simulink model "Zone_1_Zone_2_Thyristor_240Hz_R2022b"  (R2022b)
settings: Solver=FixedStepDiscrete  StartTime=0.0  StopTime=5  FixedStep=Ts  RelTol=1e-3  EnableMultiTasking=on
undefined symbols (not defined in the file or in its folder): DiscIntNeverNeededParam, GABDA, GABDB, GBBDA, GBBDB, GPPMA, GPPMB, GPPMC, SADA, SADB, SADC, SADD, SBDA, SBDB, SBDC, SCDA, SCDB, SCDC, SCDD, SDDA, SDDB, SDDC, SDDD, SDDE, TsELEC
libraries: nesl_utility x70, fl_lib x60, ee_lib x44, eeThyristorSixPulseGenerator x2, spsPowerLib x2, eeSinusoidalMeasurement x2
(part 3 of 3)

== system Zone_1_Zone_2_Thyristor_240Hz_R2022b/Subsystem16 ==
  Inductor1 : fl_lib/Electrical/Electrical Elements/Inductor  l=5.32e-6/2 H  r=0.32e-3/2 Ohm  g=0 1/Ohm  i_specify=off  i_priority=None  i=0 A  i_nominal_specify=off  i_nominal_unit=A  i_nominal_value=1  v_specify=off  v_priority=None  v=0 V  v_nominal_specify=off  v_nominal_unit=V  v_nominal_value=1  i_L_specify=off  i_L_priority=High  i_L=0 A  i_L_nominal_specify=off  i_L_nominal_unit=A  i_L_nominal_value=1
  Inductor2 : fl_lib/Electrical/Electrical Elements/Inductor  l=5.32e-6/2 H  r=0.32e-3/2 Ohm  g=0 1/Ohm  i_specify=off  i_priority=None  i=0 A  i_nominal_specify=off  i_nominal_unit=A  i_nominal_value=1  v_specify=off  v_priority=None  v=0 V  v_nominal_specify=off  v_nominal_unit=V  v_nominal_value=1  i_L_specify=off  i_L_priority=High  i_L=0 A  i_L_nominal_specify=off  i_L_nominal_unit=A  i_L_nominal_value=1
  "+ " : PMIOPort  Side=Left
  + : PMIOPort  Port=2  Side=Right
  - : PMIOPort  Port=3  Side=Left
  "- " : PMIOPort  Port=4  Side=Right
  connections:
  Inductor1/RConn1 -- "- "/RConn1
  Inductor2/RConn1 -- +/RConn1
  Inductor2/LConn1 -- "+ "/RConn1
  Inductor1/LConn1 -- -/RConn1

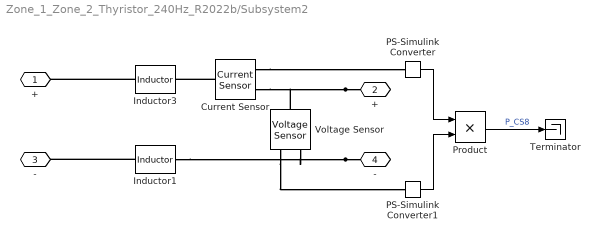
== system Zone_1_Zone_2_Thyristor_240Hz_R2022b/Subsystem2 ==
  Current Sensor : fl_lib/Electrical/Electrical Sensors/Current Sensor
  Inductor1 : fl_lib/Electrical/Electrical Elements/Inductor  l=5e-6/2 H  r=0.2e-3/2 Ohm  g=0 1/Ohm  i_specify=off  i_priority=None  i=0 A  i_nominal_specify=off  i_nominal_unit=A  i_nominal_value=1  v_specify=off  v_priority=None  v=0 V  v_nominal_specify=off  v_nominal_unit=V  v_nominal_value=1  i_L_specify=off  i_L_priority=High  i_L=0 A  i_L_nominal_specify=off  i_L_nominal_unit=A  i_L_nominal_value=1
  Inductor3 : fl_lib/Electrical/Electrical Elements/Inductor  l=5e-6/2 H  r=0.2e-3/2 Ohm  g=0 1/Ohm  i_specify=off  i_priority=None  i=0 A  i_nominal_specify=off  i_nominal_unit=A  i_nominal_value=1  v_specify=off  v_priority=None  v=0 V  v_nominal_specify=off  v_nominal_unit=V  v_nominal_value=1  i_L_specify=off  i_L_priority=High  i_L=0 A  i_L_nominal_specify=off  i_L_nominal_unit=A  i_L_nominal_value=1
  PS-Simulink Converter : nesl_utility/PS-Simulink Converter  PhysicalDomain=network_engine_domain  SubClassName=ps_output  LeftPortType=input  RightPortType=output  PseudoPeriodic=off  Frequencies=[]  VectorFormat=1-D array  Unit=inherit  AffineConversion=off
  PS-Simulink Converter1 : nesl_utility/PS-Simulink Converter  PhysicalDomain=network_engine_domain  SubClassName=ps_output  LeftPortType=input  RightPortType=output  PseudoPeriodic=off  Frequencies=[]  VectorFormat=1-D array  Unit=inherit  AffineConversion=off
  Product : Product
  Terminator : Terminator
  Voltage Sensor : fl_lib/Electrical/Electrical Sensors/Voltage Sensor
  "+ " : PMIOPort  Side=Left
  + : PMIOPort  Port=2  Side=Right
  - : PMIOPort  Port=3  Side=Left
  "- " : PMIOPort  Port=4  Side=Right
  wires:
  PS-Simulink Converter1/1 -> Product/2
  PS-Simulink Converter/1 -> Product/1
  Product/1 -> Terminator/1  "P_CS8"
  connections:
  Current Sensor/RConn1 -- PS-Simulink Converter/LConn1
  Voltage Sensor/RConn1 -- PS-Simulink Converter1/LConn1
  "- "/RConn1 -- Voltage Sensor/RConn2 -- Inductor1/RConn1
  +/RConn1 -- Voltage Sensor/LConn1 -- Current Sensor/RConn2
  Current Sensor/LConn1 -- Inductor3/RConn1
  Inductor3/LConn1 -- "+ "/RConn1
  Inductor1/LConn1 -- -/RConn1

== system Zone_1_Zone_2_Thyristor_240Hz_R2022b/Subsystem3 ==
  Inductor1 : fl_lib/Electrical/Electrical Elements/Inductor  l=2.63e-6/2 H  r=0.16e-3/2 Ohm  g=0 1/Ohm  i_specify=off  i_priority=None  i=0 A  i_nominal_specify=off  i_nominal_unit=A  i_nominal_value=1  v_specify=off  v_priority=None  v=0 V  v_nominal_specify=off  v_nominal_unit=V  v_nominal_value=1  i_L_specify=off  i_L_priority=High  i_L=0 A  i_L_nominal_specify=off  i_L_nominal_unit=A  i_L_nominal_value=1
  Inductor3 : fl_lib/Electrical/Electrical Elements/Inductor  l=2.63e-6/2 H  r=0.16e-3/2 Ohm  g=0 1/Ohm  i_specify=off  i_priority=None  i=0 A  i_nominal_specify=off  i_nominal_unit=A  i_nominal_value=1  v_specify=off  v_priority=None  v=0 V  v_nominal_specify=off  v_nominal_unit=V  v_nominal_value=1  i_L_specify=off  i_L_priority=High  i_L=0 A  i_L_nominal_specify=off  i_L_nominal_unit=A  i_L_nominal_value=1
  "+ " : PMIOPort  Side=Left
  + : PMIOPort  Port=2  Side=Right
  - : PMIOPort  Port=3  Side=Left
  "- " : PMIOPort  Port=4  Side=Right
  connections:
  Inductor1/RConn1 -- "- "/RConn1
  Inductor3/RConn1 -- +/RConn1
  Inductor3/LConn1 -- "+ "/RConn1
  Inductor1/LConn1 -- -/RConn1

== system Zone_1_Zone_2_Thyristor_240Hz_R2022b/Subsystem4 ==
  In1 : Inport
  Demux1 : Demux  Outputs=[9 1 1]
  Terminator : Terminator
  breaker status : Subsystem
  tag scope: Z1_Efd=global
  wires:
  Demux1/1 -> breaker status/1(In1)  "breakers"
  Demux1/3 -> Terminator/1
  Demux1/2 -> [Z1_Efd]  "Efd"
  In1/1 -> Demux1/1

== system Zone_1_Zone_2_Thyristor_240Hz_R2022b/Subsystem5 ==
  Inductor1 : fl_lib/Electrical/Electrical Elements/Inductor  l=5.32e-6/2 H  r=0.32e-3/2 Ohm  g=0 1/Ohm  i_specify=off  i_priority=None  i=0 A  i_nominal_specify=off  i_nominal_unit=A  i_nominal_value=1  v_specify=off  v_priority=None  v=0 V  v_nominal_specify=off  v_nominal_unit=V  v_nominal_value=1  i_L_specify=off  i_L_priority=High  i_L=0 A  i_L_nominal_specify=off  i_L_nominal_unit=A  i_L_nominal_value=1
  Inductor2 : fl_lib/Electrical/Electrical Elements/Inductor  l=5.32e-6/2 H  r=0.32e-3/2 Ohm  g=0 1/Ohm  i_specify=off  i_priority=None  i=0 A  i_nominal_specify=off  i_nominal_unit=A  i_nominal_value=1  v_specify=off  v_priority=None  v=0 V  v_nominal_specify=off  v_nominal_unit=V  v_nominal_value=1  i_L_specify=off  i_L_priority=High  i_L=0 A  i_L_nominal_specify=off  i_L_nominal_unit=A  i_L_nominal_value=1
  "+ " : PMIOPort  Side=Left
  + : PMIOPort  Port=2  Side=Right
  - : PMIOPort  Port=3  Side=Left
  "- " : PMIOPort  Port=4  Side=Right
  connections:
  Inductor1/LConn1 -- -/RConn1
  Inductor2/LConn1 -- "+ "/RConn1
  Inductor2/RConn1 -- +/RConn1
  Inductor1/RConn1 -- "- "/RConn1

== system Zone_1_Zone_2_Thyristor_240Hz_R2022b/Subsystem6 ==
  In1 : Inport
  Demux2 : Demux  Outputs=[14 1 1 1]
  Terminator1 : Terminator
  breaker status1 : Subsystem
  tag scope: PMM=global, Z2_Efd=global
  wires:
  Demux2/1 -> breaker status1/1(In1)  "breakers"
  Demux2/3 -> Terminator1/1
  Demux2/4 -> [PMM]
  Demux2/2 -> [Z2_Efd]  "Efd"
  In1/1 -> Demux2/1

== system Zone_1_Zone_2_Thyristor_240Hz_R2022b/Subsystem7 ==
  Simulink-PS Converter : nesl_utility/Simulink-PS Converter  PhysicalDomain=network_engine_domain  SubClassName=ps_input  LeftPortType=input  RightPortType=output  PseudoPeriodic=off  Frequencies=[]  NoiseDistribution=none  NoiseParameters=[]  Unit=1  AffineConversion=off  FilteringAndDerivatives=provide  SimscapeFilterOrder=1  InputFilterTimeConstant=0.001  UdotUserProvided=0
  Variable Resistor : fl_lib/Electrical/Electrical Elements/Variable Resistor  Rmin=0 Ohm  i_specify=off  i_priority=None  i=0 A  i_nominal_specify=off  i_nominal_unit=A  i_nominal_value=1  v_specify=off  v_priority=None  v=0 V  v_nominal_specify=off  v_nominal_unit=V  v_nominal_value=1
  + : PMIOPort  Side=Left
  - : PMIOPort  Port=2  Side=Left
  wires:
  [PMM] -> Simulink-PS Converter/1
  connections:
  Simulink-PS Converter/RConn1 -- Variable Resistor/LConn1
  Variable Resistor/LConn2 -- +/RConn1
  Variable Resistor/RConn1 -- -/RConn1

== system Zone_1_Zone_2_Thyristor_240Hz_R2022b/Subsystem8 ==
  Inductor1 : fl_lib/Electrical/Electrical Elements/Inductor  l=2.63e-6/2 H  r=0.16e-3/2 Ohm  g=0 1/Ohm  i_specify=off  i_priority=None  i=0 A  i_nominal_specify=off  i_nominal_unit=A  i_nominal_value=1  v_specify=off  v_priority=None  v=0 V  v_nominal_specify=off  v_nominal_unit=V  v_nominal_value=1  i_L_specify=off  i_L_priority=High  i_L=0 A  i_L_nominal_specify=off  i_L_nominal_unit=A  i_L_nominal_value=1
  Inductor3 : fl_lib/Electrical/Electrical Elements/Inductor  l=2.63e-6/2 H  r=0.16e-3/2 Ohm  g=0 1/Ohm  i_specify=off  i_priority=None  i=0 A  i_nominal_specify=off  i_nominal_unit=A  i_nominal_value=1  v_specify=off  v_priority=None  v=0 V  v_nominal_specify=off  v_nominal_unit=V  v_nominal_value=1  i_L_specify=off  i_L_priority=High  i_L=0 A  i_L_nominal_specify=off  i_L_nominal_unit=A  i_L_nominal_value=1
  "+ " : PMIOPort  Side=Left
  + : PMIOPort  Port=2  Side=Right
  - : PMIOPort  Port=3  Side=Left
  "- " : PMIOPort  Port=4  Side=Right
  connections:
  Inductor1/LConn1 -- -/RConn1
  Inductor3/LConn1 -- "+ "/RConn1
  Inductor3/RConn1 -- +/RConn1
  Inductor1/RConn1 -- "- "/RConn1

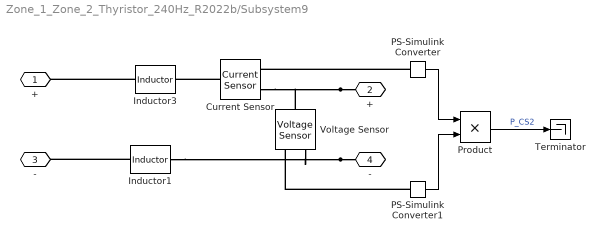
== system Zone_1_Zone_2_Thyristor_240Hz_R2022b/Subsystem9 ==
  Current Sensor : fl_lib/Electrical/Electrical Sensors/Current Sensor
  Inductor1 : fl_lib/Electrical/Electrical Elements/Inductor  l=3.47e-6/2 H  r=0.21e-3/2 Ohm  g=0 1/Ohm  i_specify=off  i_priority=None  i=0 A  i_nominal_specify=off  i_nominal_unit=A  i_nominal_value=1  v_specify=off  v_priority=None  v=0 V  v_nominal_specify=off  v_nominal_unit=V  v_nominal_value=1  i_L_specify=off  i_L_priority=High  i_L=0 A  i_L_nominal_specify=off  i_L_nominal_unit=A  i_L_nominal_value=1
  Inductor3 : fl_lib/Electrical/Electrical Elements/Inductor  l=3.47e-6/2 H  r=0.21e-3/2 Ohm  g=0 1/Ohm  i_specify=off  i_priority=None  i=0 A  i_nominal_specify=off  i_nominal_unit=A  i_nominal_value=1  v_specify=off  v_priority=None  v=0 V  v_nominal_specify=off  v_nominal_unit=V  v_nominal_value=1  i_L_specify=off  i_L_priority=High  i_L=0 A  i_L_nominal_specify=off  i_L_nominal_unit=A  i_L_nominal_value=1
  PS-Simulink Converter : nesl_utility/PS-Simulink Converter  PhysicalDomain=network_engine_domain  SubClassName=ps_output  LeftPortType=input  RightPortType=output  PseudoPeriodic=off  Frequencies=[]  VectorFormat=1-D array  Unit=inherit  AffineConversion=off
  PS-Simulink Converter1 : nesl_utility/PS-Simulink Converter  PhysicalDomain=network_engine_domain  SubClassName=ps_output  LeftPortType=input  RightPortType=output  PseudoPeriodic=off  Frequencies=[]  VectorFormat=1-D array  Unit=inherit  AffineConversion=off
  Product : Product
  Terminator : Terminator
  Voltage Sensor : fl_lib/Electrical/Electrical Sensors/Voltage Sensor
  "+ " : PMIOPort  Side=Left
  + : PMIOPort  Port=2  Side=Right
  - : PMIOPort  Port=3  Side=Left
  "- " : PMIOPort  Port=4  Side=Right
  wires:
  Product/1 -> Terminator/1  "P_CS2"
  PS-Simulink Converter1/1 -> Product/2
  PS-Simulink Converter/1 -> Product/1
  connections:
  PS-Simulink Converter1/LConn1 -- Voltage Sensor/RConn1
  PS-Simulink Converter/LConn1 -- Current Sensor/RConn1
  +/RConn1 -- Voltage Sensor/LConn1 -- Current Sensor/RConn2
  Current Sensor/LConn1 -- Inductor3/RConn1
  "- "/RConn1 -- Voltage Sensor/RConn2 -- Inductor1/RConn1
  Inductor1/LConn1 -- -/RConn1
  Inductor3/LConn1 -- "+ "/RConn1

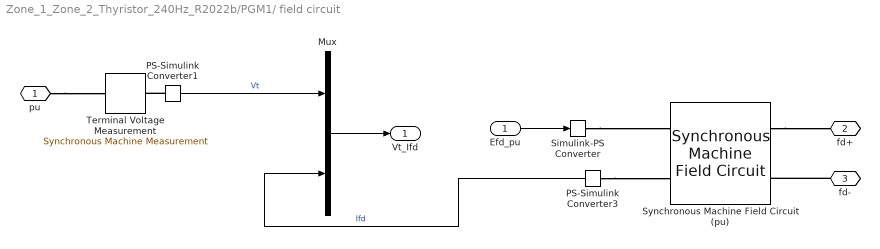
== system Zone_1_Zone_2_Thyristor_240Hz_R2022b/PGM1/ field circuit ==
  Efd_pu : Inport
  Mux : Mux  Inputs=2
  PS-Simulink Converter1 : nesl_utility/PS-Simulink Converter  PhysicalDomain=network_engine_domain  SubClassName=ps_output  LeftPortType=input  RightPortType=output  PseudoPeriodic=off  Frequencies=[]  VectorFormat=1-D array  Unit=inherit  AffineConversion=off
  PS-Simulink Converter3 : nesl_utility/PS-Simulink Converter  PhysicalDomain=network_engine_domain  SubClassName=ps_output  LeftPortType=input  RightPortType=output  PseudoPeriodic=off  Frequencies=[]  VectorFormat=1-D array  Unit=inherit  AffineConversion=off
  Simulink-PS Converter : nesl_utility/Simulink-PS Converter  PhysicalDomain=network_engine_domain  SubClassName=ps_input  LeftPortType=input  RightPortType=output  PseudoPeriodic=off  Frequencies=[]  NoiseDistribution=none  NoiseParameters=[]  Unit=1  AffineConversion=off  FilteringAndDerivatives=zero  SimscapeFilterOrder=1  InputFilterTimeConstant=0.001  UdotUserProvided=0
  Synchronous Machine Field Circuit (pu) : ee_lib/Electromechanical/Synchronous/Synchronous Machine Field Circuit  unit_option=ee.enum.unit.pu  SRated=45e6 V*A  FRated=240 Hz  fieldCircuitParameterization_option=ee.enum.sm.fieldparameterization.current  baseEfd=92.95 V  baseIfd=200 A  parameterization_option=ee.enum.sm.parameterization.standard  Ladu=1.66  Rfd=0.0006  Xl=0.08  Xd=1.352  Xdd=0.296  Xddd=0.148  d_option=ee.enum.circuit.open  Td0d=4.141 s  Tdd=1.3260 s  Td0dd=0.027 s  Tddd=0.0230 s
      settings: LogSimulationData=on  InternalSimscapePortConfiguration="{\"Bottom\":[],\"Left\":[{\"id\":\"Efd_pu\",\"label\":\"Efd_pu\",\"type\":\"input\"},{\"id\":\"Ifd_pu\",\"label\":\"Ifd_pu\",\"type\":\"output\"}],\"Right\":[{\"id\":\"fd_p\",\"label\":\"fd+\",\"type\":\"foundation.electrical.electrical\"},{\"id\":\"fd_n\",\"label\":\"fd-\",\"type\":\"foundation.electrical.electrical\"}],\"Top\":[]}"
  Terminal Voltage Measurement : ee_lib/Electromechanical/Synchronous/Synchronous Machine Measurement  output_idx=14
      settings: LogSimulationData=on  InternalSimscapePortConfiguration="{\"Bottom\":[],\"Left\":[{\"id\":\"pu_input\",\"label\":\"pu\",\"type\":\"input\"}],\"Right\":[{\"id\":\"pu_output\",\"label\":\"o\",\"type\":\"output\"}],\"Top\":[]}"
  pu : PMIOPort  Side=Left
  fd+ : PMIOPort  Port=2  Side=Right
  fd- : PMIOPort  Port=3  Side=Right
  Vt_Ifd : Outport
  wires:
  Mux/1 -> Vt_Ifd/1
  PS-Simulink Converter3/1 -> Mux/2  "Ifd"
  PS-Simulink Converter1/1 -> Mux/1  "Vt"
  Efd_pu/1 -> Simulink-PS Converter/1
  connections:
  PS-Simulink Converter1/LConn1 -- Terminal Voltage Measurement/RConn1
  pu/RConn1 -- Terminal Voltage Measurement/LConn1
  Simulink-PS Converter/RConn1 -- Synchronous Machine Field Circuit (pu)/LConn1
  PS-Simulink Converter3/LConn1 -- Synchronous Machine Field Circuit (pu)/LConn2
  Synchronous Machine Field Circuit (pu)/RConn1 -- fd+/RConn1
  fd-/RConn1 -- Synchronous Machine Field Circuit (pu)/RConn2

== system Zone_1_Zone_2_Thyristor_240Hz_R2022b/PGM1/Gate driver ==
  S : Inport
  Demux : Demux  Outputs=6
  Simulink-PS Converter{,1..5} (6 alike) : nesl_utility/Simulink-PS Converter  PhysicalDomain=network_engine_domain  SubClassName=ps_input  LeftPortType=input  RightPortType=output  PseudoPeriodic=off  Frequencies=[]  NoiseDistribution=none  NoiseParameters=[]  Unit=1  AffineConversion=off  FilteringAndDerivatives=zero  SimscapeFilterOrder=1  InputFilterTimeConstant=0.001  UdotUserProvided=0
  Six-Pulse Gate Multiplexer : ee_lib/Semiconductors & Converters/Converters/Six-Pulse Gate Multiplexer  port_option=ee.enum.controlport.ps
  G : PMIOPort  Side=Right
  wires:
  Demux/1 -> Simulink-PS Converter/1
  Demux/5 -> Simulink-PS Converter4/1
  Demux/2 -> Simulink-PS Converter1/1
  Demux/4 -> Simulink-PS Converter3/1
  S/1 -> Demux/1
  Demux/3 -> Simulink-PS Converter2/1
  Demux/6 -> Simulink-PS Converter5/1
  connections:
  Six-Pulse Gate Multiplexer/RConn1 -- G/RConn1
  Simulink-PS Converter4/RConn1 -- Six-Pulse Gate Multiplexer/LConn5
  Simulink-PS Converter/RConn1 -- Six-Pulse Gate Multiplexer/LConn1
  Simulink-PS Converter3/RConn1 -- Six-Pulse Gate Multiplexer/LConn4
  Simulink-PS Converter2/RConn1 -- Six-Pulse Gate Multiplexer/LConn3
  Simulink-PS Converter1/RConn1 -- Six-Pulse Gate Multiplexer/LConn2
  Simulink-PS Converter5/RConn1 -- Six-Pulse Gate Multiplexer/LConn6

== system Zone_1_Zone_2_Thyristor_240Hz_R2022b/PGM1/Sensing current ==
  Current Sensor : ee_lib/Sensors & Transducers/Current Sensor (Three-Phase)
  PS-Simulink Converter : nesl_utility/PS-Simulink Converter  PhysicalDomain=network_engine_domain  SubClassName=ps_output  LeftPortType=input  RightPortType=output  PseudoPeriodic=off  Frequencies=[]  VectorFormat=1-D array  Unit=A  AffineConversion=off
  1~ : PMIOPort  Side=Left
  2~ : PMIOPort  Port=2  Side=Right
  tag scope: Iabc1=global
  wires:
  PS-Simulink Converter/1 -> [Iabc1]
  connections:
  2~/RConn1 -- Current Sensor/RConn2
  PS-Simulink Converter/LConn1 -- Current Sensor/RConn1
  Current Sensor/LConn1 -- 1~/RConn1

== system Zone_1_Zone_2_Thyristor_240Hz_R2022b/PGM1/Sensing voltage ==
  PS-Simulink Converter : nesl_utility/PS-Simulink Converter  PhysicalDomain=network_engine_domain  SubClassName=ps_output  LeftPortType=input  RightPortType=output  PseudoPeriodic=off  Frequencies=[]  VectorFormat=1-D array  Unit=V  AffineConversion=off
  Phase Voltage Sensor : ee_lib/Sensors & Transducers/Phase Voltage Sensor (Three-Phase)
  ~2 : PMIOPort  Side=Right
  ~1 : PMIOPort  Port=2  Side=Left
  tag scope: Vabc1=global
  wires:
  PS-Simulink Converter/1 -> [Vabc1]
  connections:
  Phase Voltage Sensor/LConn1 -- ~1/RConn1
  Phase Voltage Sensor/RConn2 -- ~2/RConn1
  PS-Simulink Converter/LConn1 -- Phase Voltage Sensor/RConn1

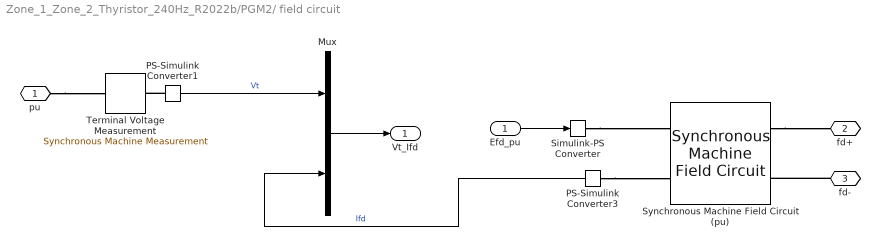
== system Zone_1_Zone_2_Thyristor_240Hz_R2022b/PGM2/ field circuit ==
  Efd_pu : Inport
  Mux : Mux  Inputs=2
  PS-Simulink Converter1 : nesl_utility/PS-Simulink Converter  PhysicalDomain=network_engine_domain  SubClassName=ps_output  LeftPortType=input  RightPortType=output  PseudoPeriodic=off  Frequencies=[]  VectorFormat=1-D array  Unit=inherit  AffineConversion=off
  PS-Simulink Converter3 : nesl_utility/PS-Simulink Converter  PhysicalDomain=network_engine_domain  SubClassName=ps_output  LeftPortType=input  RightPortType=output  PseudoPeriodic=off  Frequencies=[]  VectorFormat=1-D array  Unit=inherit  AffineConversion=off
  Simulink-PS Converter : nesl_utility/Simulink-PS Converter  PhysicalDomain=network_engine_domain  SubClassName=ps_input  LeftPortType=input  RightPortType=output  PseudoPeriodic=off  Frequencies=[]  NoiseDistribution=none  NoiseParameters=[]  Unit=1  AffineConversion=off  FilteringAndDerivatives=zero  SimscapeFilterOrder=1  InputFilterTimeConstant=0.001  UdotUserProvided=0
  Synchronous Machine Field Circuit (pu) : ee_lib/Electromechanical/Synchronous/Synchronous Machine Field Circuit  unit_option=ee.enum.unit.pu  SRated=45e6 V*A  FRated=240 Hz  fieldCircuitParameterization_option=ee.enum.sm.fieldparameterization.current  baseEfd=92.95 V  baseIfd=200 A  parameterization_option=ee.enum.sm.parameterization.standard  Ladu=1.66  Rfd=0.0006  Xl=0.08  Xd=1.352  Xdd=0.296  Xddd=0.148  d_option=ee.enum.circuit.open  Td0d=4.141 s  Tdd=1.3260 s  Td0dd=0.027 s  Tddd=0.0230 s
      settings: LogSimulationData=on  InternalSimscapePortConfiguration="{\"Bottom\":[],\"Left\":[{\"id\":\"Efd_pu\",\"label\":\"Efd_pu\",\"type\":\"input\"},{\"id\":\"Ifd_pu\",\"label\":\"Ifd_pu\",\"type\":\"output\"}],\"Right\":[{\"id\":\"fd_p\",\"label\":\"fd+\",\"type\":\"foundation.electrical.electrical\"},{\"id\":\"fd_n\",\"label\":\"fd-\",\"type\":\"foundation.electrical.electrical\"}],\"Top\":[]}"
  Terminal Voltage Measurement : ee_lib/Electromechanical/Synchronous/Synchronous Machine Measurement  output_idx=14
      settings: LogSimulationData=on  InternalSimscapePortConfiguration="{\"Bottom\":[],\"Left\":[{\"id\":\"pu_input\",\"label\":\"pu\",\"type\":\"input\"}],\"Right\":[{\"id\":\"pu_output\",\"label\":\"o\",\"type\":\"output\"}],\"Top\":[]}"
  pu : PMIOPort  Side=Left
  fd+ : PMIOPort  Port=2  Side=Right
  fd- : PMIOPort  Port=3  Side=Right
  Vt_Ifd : Outport
  wires:
  Efd_pu/1 -> Simulink-PS Converter/1
  PS-Simulink Converter1/1 -> Mux/1  "Vt"
  PS-Simulink Converter3/1 -> Mux/2  "Ifd"
  Mux/1 -> Vt_Ifd/1
  connections:
  fd-/RConn1 -- Synchronous Machine Field Circuit (pu)/RConn2
  Synchronous Machine Field Circuit (pu)/RConn1 -- fd+/RConn1
  PS-Simulink Converter3/LConn1 -- Synchronous Machine Field Circuit (pu)/LConn2
  Simulink-PS Converter/RConn1 -- Synchronous Machine Field Circuit (pu)/LConn1
  pu/RConn1 -- Terminal Voltage Measurement/LConn1
  PS-Simulink Converter1/LConn1 -- Terminal Voltage Measurement/RConn1

== system Zone_1_Zone_2_Thyristor_240Hz_R2022b/PGM2/Gate driver ==
  S : Inport
  Demux : Demux  Outputs=6
  Simulink-PS Converter{,1..5} (6 alike) : nesl_utility/Simulink-PS Converter  PhysicalDomain=network_engine_domain  SubClassName=ps_input  LeftPortType=input  RightPortType=output  PseudoPeriodic=off  Frequencies=[]  NoiseDistribution=none  NoiseParameters=[]  Unit=1  AffineConversion=off  FilteringAndDerivatives=zero  SimscapeFilterOrder=1  InputFilterTimeConstant=0.001  UdotUserProvided=0
  Six-Pulse Gate Multiplexer : ee_lib/Semiconductors & Converters/Converters/Six-Pulse Gate Multiplexer  port_option=ee.enum.controlport.ps
  G : PMIOPort  Side=Right
  wires:
  Demux/6 -> Simulink-PS Converter5/1
  Demux/3 -> Simulink-PS Converter2/1
  S/1 -> Demux/1
  Demux/4 -> Simulink-PS Converter3/1
  Demux/2 -> Simulink-PS Converter1/1
  Demux/5 -> Simulink-PS Converter4/1
  Demux/1 -> Simulink-PS Converter/1
  connections:
  Simulink-PS Converter5/RConn1 -- Six-Pulse Gate Multiplexer/LConn6
  Simulink-PS Converter1/RConn1 -- Six-Pulse Gate Multiplexer/LConn2
  Simulink-PS Converter2/RConn1 -- Six-Pulse Gate Multiplexer/LConn3
  Simulink-PS Converter3/RConn1 -- Six-Pulse Gate Multiplexer/LConn4
  Simulink-PS Converter/RConn1 -- Six-Pulse Gate Multiplexer/LConn1
  Simulink-PS Converter4/RConn1 -- Six-Pulse Gate Multiplexer/LConn5
  Six-Pulse Gate Multiplexer/RConn1 -- G/RConn1

== system Zone_1_Zone_2_Thyristor_240Hz_R2022b/PGM2/Sensing current ==
  Current Sensor : ee_lib/Sensors & Transducers/Current Sensor (Three-Phase)
  PS-Simulink Converter : nesl_utility/PS-Simulink Converter  PhysicalDomain=network_engine_domain  SubClassName=ps_output  LeftPortType=input  RightPortType=output  PseudoPeriodic=off  Frequencies=[]  VectorFormat=1-D array  Unit=A  AffineConversion=off
  1~ : PMIOPort  Side=Left
  2~ : PMIOPort  Port=2  Side=Right
  tag scope: Iabc=global
  wires:
  PS-Simulink Converter/1 -> [Iabc]
  connections:
  Current Sensor/LConn1 -- 1~/RConn1
  PS-Simulink Converter/LConn1 -- Current Sensor/RConn1
  2~/RConn1 -- Current Sensor/RConn2

== system Zone_1_Zone_2_Thyristor_240Hz_R2022b/PGM2/Sensing voltage ==
  PS-Simulink Converter : nesl_utility/PS-Simulink Converter  PhysicalDomain=network_engine_domain  SubClassName=ps_output  LeftPortType=input  RightPortType=output  PseudoPeriodic=off  Frequencies=[]  VectorFormat=1-D array  Unit=V  AffineConversion=off
  Phase Voltage Sensor : ee_lib/Sensors & Transducers/Phase Voltage Sensor (Three-Phase)
  ~2 : PMIOPort  Side=Right
  ~1 : PMIOPort  Port=2  Side=Left
  tag scope: Vabc=global
  wires:
  PS-Simulink Converter/1 -> [Vabc]
  connections:
  PS-Simulink Converter/LConn1 -- Phase Voltage Sensor/RConn1
  Phase Voltage Sensor/RConn2 -- ~2/RConn1
  Phase Voltage Sensor/LConn1 -- ~1/RConn1

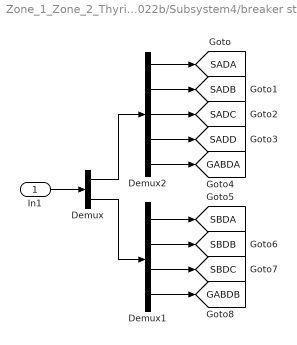
== system Zone_1_Zone_2_Thyristor_240Hz_R2022b/Subsystem4/breaker status ==
  In1 : Inport
  Demux : Demux  Outputs=[5 4]
  Demux1 : Demux
  Demux2 : Demux  Outputs=5
  tag scope: GABDA=global, GABDB=global, SADA=global, SADB=global, SADC=global, SADD=global, SBDA=global, SBDB=global, SBDC=global
  wires:
  Demux1/4 -> [GABDB]
  Demux1/3 -> [SBDC]
  Demux1/2 -> [SBDB]
  Demux1/1 -> [SBDA]
  Demux/2 -> Demux1/1
  Demux/1 -> Demux2/1
  In1/1 -> Demux/1
  Demux2/4 -> [SADD]
  Demux2/3 -> [SADC]
  Demux2/1 -> [SADA]
  Demux2/2 -> [SADB]
  Demux2/5 -> [GABDA]

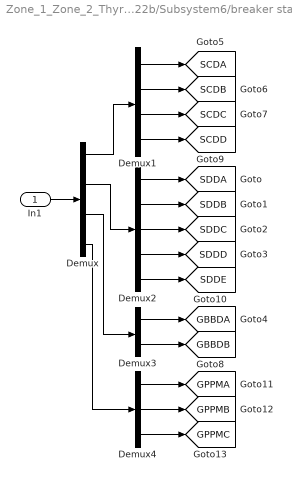
== system Zone_1_Zone_2_Thyristor_240Hz_R2022b/Subsystem6/breaker status1 ==
  In1 : Inport
  Demux : Demux  Outputs=[4 5 2 3]
  Demux1 : Demux
  Demux2 : Demux  Outputs=5
  Demux3 : Demux  Outputs=2
  Demux4 : Demux  Outputs=3
  tag scope: GBBDA=global, GBBDB=global, GPPMA=global, GPPMB=global, GPPMC=global, SCDA=global, SCDB=global, SCDC=global, SCDD=global, SDDA=global, SDDB=global, SDDC=global, SDDD=global, SDDE=global
  wires:
  Demux/4 -> Demux4/1
  Demux4/3 -> [GPPMC]
  Demux4/2 -> [GPPMB]
  Demux4/1 -> [GPPMA]
  Demux/3 -> Demux3/1
  Demux3/2 -> [GBBDB]
  Demux3/1 -> [GBBDA]
  Demux/2 -> Demux2/1
  Demux/1 -> Demux1/1
  Demux2/5 -> [SDDE]
  Demux1/4 -> [SCDD]
  Demux1/3 -> [SCDC]
  Demux1/2 -> [SCDB]
  Demux1/1 -> [SCDA]
  In1/1 -> Demux/1
  Demux2/4 -> [SDDD]
  Demux2/3 -> [SDDC]
  Demux2/1 -> [SDDA]
  Demux2/2 -> [SDDB]
